simulink model "DD20220330"  (R2021a)
settings: Solver=VariableStepAuto  StartTime=0.0  StopTime=50  RelTol=1e-3
undefined symbols (not defined in the file): A, B, g, K, L, m, tau
settings Model: Creator=jaewan  LastModifiedBy=jaewan

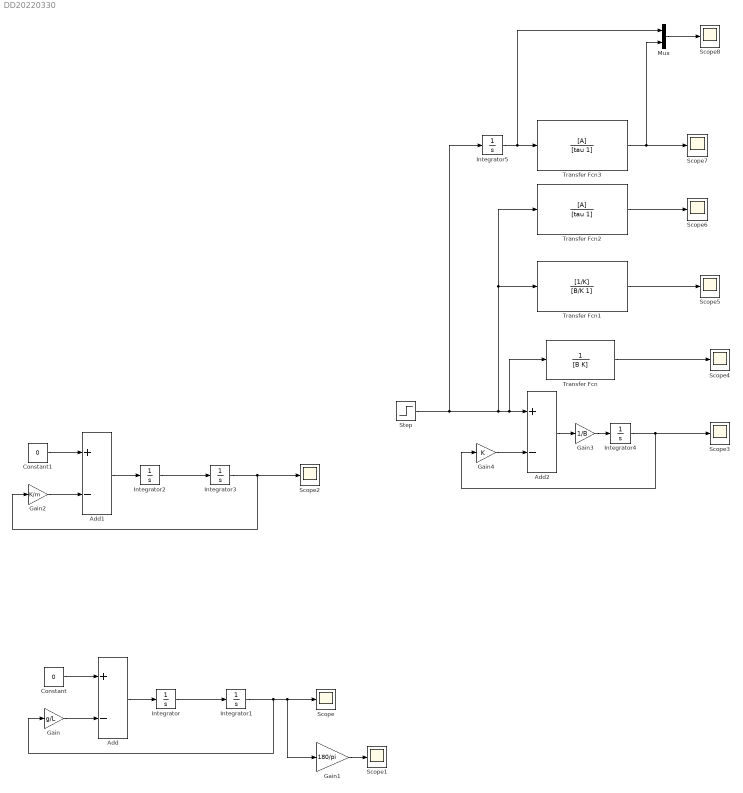
== system DD20220330 ==
  Add : Sum  Inputs=+-
  Add1 : Sum  Inputs=+-
  Add2 : Sum  Inputs=+-
  Constant : Constant  Value=0
  Constant1 : Constant  Value=0
  Gain : Gain  Gain=g/L
  Gain1 : Gain  Gain=180/pi
  Gain2 : Gain  Gain=K/m
  Gain3 : Gain  Gain=1/B
  Gain4 : Gain  Gain=K
  Integrator{,2,4..5} (4 alike) : Integrator
  Integrator1 : Integrator  InitialCondition=30*(pi/180)
  Integrator3 : Integrator  InitialCondition=1
  Mux : Mux  Inputs=2
  Scope{,1..8} (9 alike) : Scope
  Step : Step  Time=0  After=4  SampleTime=0
  Transfer Fcn : TransferFcn  Denominator=[B K]
  Transfer Fcn1 : TransferFcn  Numerator=[1/K]  Denominator=[B/K 1]
  Transfer Fcn2 : TransferFcn  Numerator=[A]  Denominator=[tau 1]
  Transfer Fcn3 : TransferFcn  Numerator=[A]  Denominator=[tau 1]
  wires:
  Integrator1/1 -> Gain/1, Gain1/1, Scope/1
  Integrator/1 -> Integrator1/1
  Gain/1 -> Add/2
  Constant/1 -> Add/1
  Add/1 -> Integrator/1
  Gain1/1 -> Scope1/1
  Integrator2/1 -> Integrator3/1
  Gain2/1 -> Add1/2
  Add1/1 -> Integrator2/1
  Constant1/1 -> Add1/1
  Integrator3/1 -> Gain2/1, Scope2/1
  Integrator4/1 -> Gain4/1, Scope3/1
  Add2/1 -> Gain3/1
  Gain3/1 -> Integrator4/1
  Gain4/1 -> Add2/2
  Transfer Fcn/1 -> Scope4/1
  Step/1 -> Integrator5/1, Transfer Fcn/1, Add2/1, Transfer Fcn2/1, Transfer Fcn1/1
  Transfer Fcn1/1 -> Scope5/1
  Transfer Fcn2/1 -> Scope6/1
  Integrator5/1 -> Mux/1, Transfer Fcn3/1
  Transfer Fcn3/1 -> Scope7/1, Mux/2
  Mux/1 -> Scope8/1
